simulink model "EOG_BCI2"  (Simulink 8.0)
settings: Solver=FixedStepDiscrete  StartTime=0.0  StopTime=1000  FixedStep=1/256  RelTol=1e-3
undefined symbols (not defined in the file or in its folder): currentCFG_EOG_BCI2_UA, UA
libraries: gtecHighspeedLib x1, gUSBamplib x1
settings Model: Creator=lab  LastModifiedBy=MA
settings DataIOCC: SignalLoggingSaveFormat=ModelDataLogs
settings DebuggingCC: FcnCallInpInsideContextMsg=UseLocalSettings  StrictBusMsg=Warning
settings GRTTargetCC: CombineOutputUpdateFcns=off  GRTInterface=on

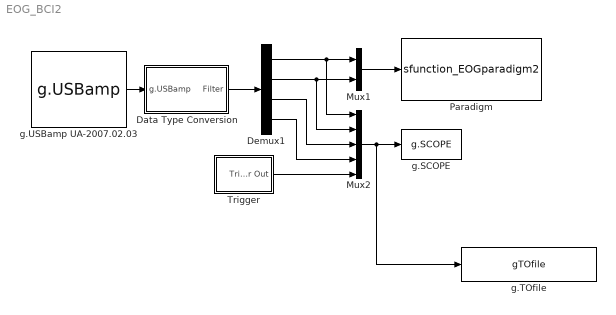
== system EOG_BCI2 ==
  Data Type Conversion : Subsystem
  Demux1 : Demux
  Mux1 : Mux  Inputs=2
  Mux2 : Mux  Inputs=5
  Paradigm : S-Function  FunctionName=sfunction_EOGparadigm2  Parameters=dofrown,doblink,dowink,dogaze,iteration  EnableBusSupport=off  mask{dofrown=on, doblink=on, dowink=on, dogaze=on, iteration=10}
      mask prompts: dofrown "frown"; doblink "blink"; dowink "wink"; dogaze "gaze"
  Trigger : Subsystem
  g.SCOPE : gtecHighspeedLib/g.SCOPE  sdf=off
  g.TOfile : S-Function  FunctionName=gTOfile  Parameters=filename, varname, filesize, blocksize  EnableBusSupport=off  mask(g.TOfile){filename=test_0807_muro, varname=y, filesize=50, blocksize=1024}
      mask prompts: varname "Variable:"; filesize "File size [MB]:"; blocksize "Block size [kB]:"
      mask help:
      | The g.TOfile block saves data as a variable into a file. If you have a very large dataset, it will be splitted into more files, so it is still possible to open it in Matlab.
      |
      | Parameter:
      | Filename - name of the file, which will be extended with a four digit number
      | Variable - name of the variable, which will be extended with a four digit number
      | File size [MB] - size of the single files in megabyte
      mask Help: web(['file:///' which('gtecHS.htm')],'-helpbrowser');
      mask Callback filename:
      | set_param(gcb, 'LinkStatus', 'none');
      | maskStr = get_param(gcb, 'MaskValues');
      | tmp = sprintf('disp(''%s'')', maskStr{1});
      | set_param(gcb, 'MaskDisplay', tmp);
      | clear maskStr tmp
      mask Callback filesize:
      | maskStr = get_param(gcb, 'MaskValues');
      | mem = memory;
      | maxMem = ((mem.MaxPossibleArrayBytes*0.99)/(1024*1024));
      | if maxMem < str2num(maskStr{3})
      |     errorStr = sprintf('File size too large!\nMaximum file size: %.0f', maxMem);
      |     errordlg(errorStr);
      | end
      | clear maskStr mem maxMem errorStr
      mask Callback blocksize:
      | maskStr = get_param(gcb, 'MaskValues');
      | fileSz = str2num(maskStr{3})*1024;
      | blockSz = str2num(maskStr{4});
      | if fileSz/2 < blockSz
      |     errorStr = sprintf('Block size to large!\nMaximum half of file size');
      |     errorDlg(errorStr);
      | end
      | clear maskStr fileSz blockSz errorStr
      mask Display: disp('test_0807_muro')
  g.USBamp UA-2007.02.03 : gUSBamplib/g.USBamp  Priority=2  cfg=currentCFG_EOG_BCI2_UA-2007.02.03.cfg  snr=UA-2007.02.03
  wires:
  g.USBamp UA-2007.02.03/1 -> Data Type Conversion/1(g.USBamp)
  Demux1/2 -> Mux1/2, Mux2/2
  Demux1/1 -> Mux1/1, Mux2/1
  Mux1/1 -> Paradigm/1
  Mux2/1 -> g.TOfile/1, g.SCOPE/1
  Demux1/3 -> Mux2/3
  Demux1/4 -> Mux2/4
  Trigger/1(Trigger Out) -> Mux2/5
  Data Type Conversion/1(Filter) -> Demux1/1

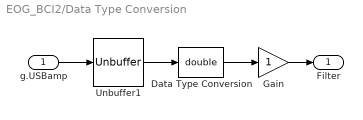
== system EOG_BCI2/Data Type Conversion ==
  g.USBamp : Inport  Priority=1
  Data Type Conversion : DataTypeConversion  OutDataTypeStr=double
  Gain : Gain  SampleTime=1/256  SaturateOnIntegerOverflow=on  OutDataTypeStr=Inherit: Same as input  ParamDataTypeStr=Inherit: Same as input
  Unbuffer1 : Unbuffer
  Filter : Outport
  wires:
  Data Type Conversion/1 -> Gain/1
  Unbuffer1/1 -> Data Type Conversion/1
  Gain/1 -> Filter/1
  g.USBamp/1 -> Unbuffer1/1

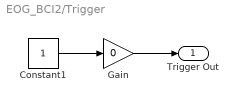
== system EOG_BCI2/Trigger ==
  Constant1 : Constant
  Gain : Gain  Gain=0  SaturateOnIntegerOverflow=on  OutDataTypeStr=Inherit: Same as input  ParamDataTypeStr=Inherit: Same as input
  Trigger Out : Outport
  wires:
  Constant1/1 -> Gain/1
  Gain/1 -> Trigger Out/1
